simulink model "simu2"  (R2024b)
settings: Solver=VariableStepAuto  StartTime=0.0  StopTime=10.0  RelTol=1e-3
values from neighbouring files (symbols this model uses):
  b = 10    [PID.m]    (also in t2.m = 0.5)
  J = 9.99 *(10^-6)    (= 9.99e-06)    [BallBeamSys.m]    (also in t2.m = 2)
  Kb = 0.1    [t2.m]
  Kt = 10    [t2.m]
  Ra = 1    [t2.m]
settings Model: Creator=Faizy  LastModifiedBy=Faizy

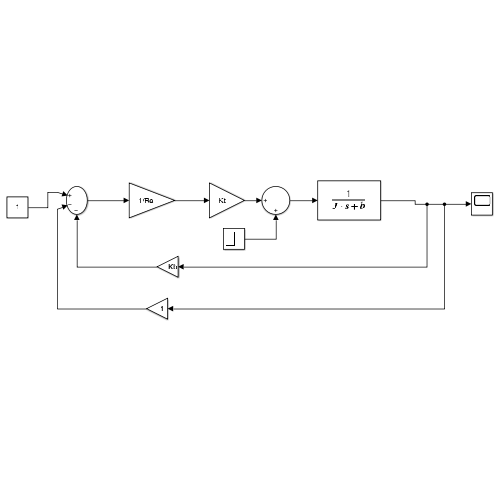
[thumbnail: Simulink's stored preview of the top-level diagram]
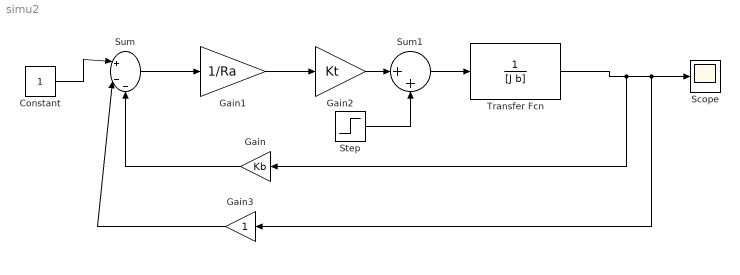
== system simu2 ==
  Constant : Constant
  Gain : Gain  Gain=Kb
  Gain1 : Gain  Gain=1/Ra
  Gain2 : Gain  Gain=Kt
  Gain3 : Gain
  Scope : Scope
  Step : Step  SampleTime=0
  Sum : Sum  Inputs=|+--
  Sum1 : Sum  Inputs=|++
  Transfer Fcn : TransferFcn  Denominator=[J b]
  wires:
  Sum/1 -> Gain1/1
  Gain1/1 -> Gain2/1
  Gain2/1 -> Sum1/1
  Sum1/1 -> Transfer Fcn/1
  Transfer Fcn/1 -> Gain/1, Gain3/1, Scope/1
  Step/1 -> Sum1/2
  Constant/1 -> Sum/1
  Gain/1 -> Sum/3
  Gain3/1 -> Sum/2
